simulink model "L5_2_G13_sim"  (R2024b)
settings: Solver=ode23tb  StartTime=0.0  StopTime=0.2  MaxStep=1/(fpwm_inv/200)  RelTol=1e-3
undefined symbols (not defined in the file): Cdc, deltafi, fac, Kii, Kivdc, Kpi, Kpvdc, Lfac, m_inv, Pac, Pdc, QCac, QLac, Rdc, Rdcmax, Udc, Vac, Vdcref, XLf
libraries: spsSeriesRLCBranchLib x6, spsThreePhaseVIMeasurementLib x3, spsCurrentMeasurementLib x2, spsabctodq0Lib x2, spsIdealSwitchLib x1, spsPLL3phLib x1, spsdq0toabcLib x1, spsPWMGenerator2LevelLib x1, spsMeanLib x1, spsPower3phInstantaneousLib x1, spsThreePhaseSourceLib x1, spsThreePhaseParallelRLCLoadLib x1
settings Model: Creator=franc  LastModifiedBy=franc

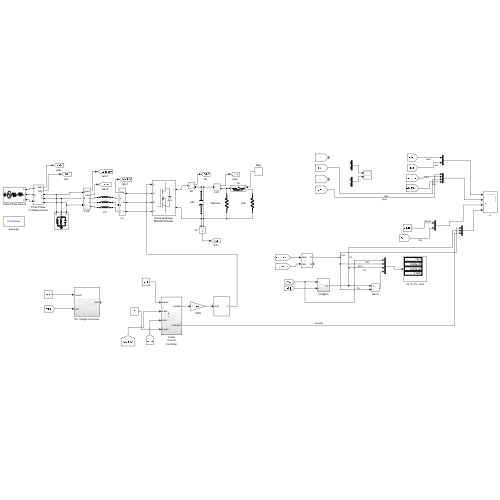
[thumbnail: Simulink's stored preview of the top-level diagram]
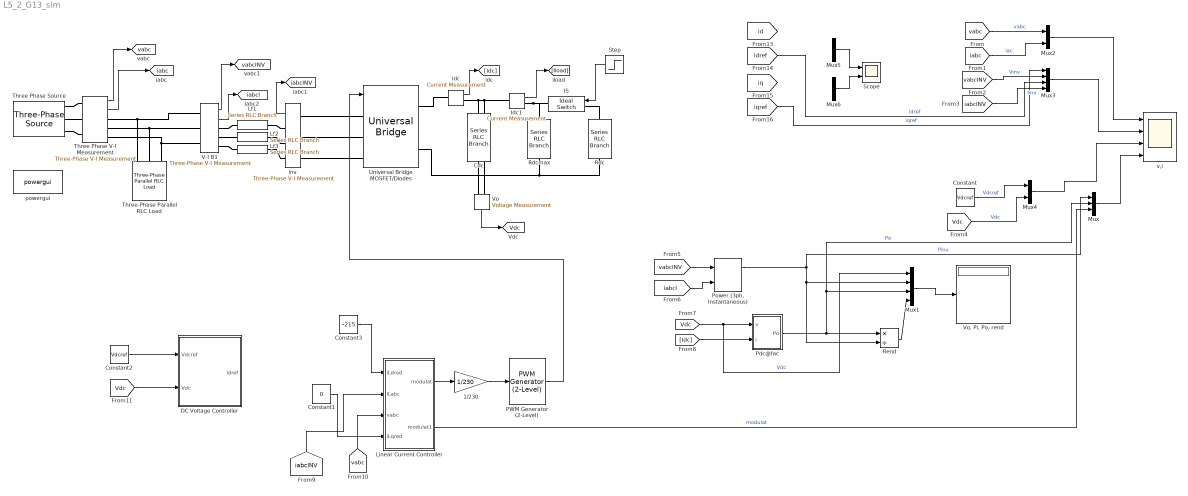
== system L5_2_G13_sim ==
  1/230 : Gain  Gain=1/230
  Cdc : spsSeriesRLCBranchLib/Series RLC Branch  LConnTagsString=__new0  RConnTagsString=__new0  BranchType=C  Resistance=1  Inductance=1e-3  SetiL0=off  InitialCurrent=0  Capacitance=Cdc  Setx0=on  InitialVoltage=0.95*Udc  Measurements=None
  Constant : Constant  Value=Vdcref
  Constant1 : Constant  Value=0
  Constant2 : Constant  Value=Vdcref
  Constant3 : Constant  Value=-215
  DC Voltage Controller : Subsystem
  IS : spsIdealSwitchLib/Ideal Switch  Ron=0.001  Lon=0  IC=0  Rs=1e5  Cs=inf  Measurements=off
  Idc : spsCurrentMeasurementLib/Current Measurement  PhasorSimulation=off  OutputType=Complex  PSBequivalent=0
  Idc1 : spsCurrentMeasurementLib/Current Measurement  PhasorSimulation=off  OutputType=Complex  PSBequivalent=0
  Lf1 : spsSeriesRLCBranchLib/Series RLC Branch  LConnTagsString=__new0  RConnTagsString=__new0  BranchType=L  Resistance=1  Inductance=Lfac  SetiL0=off  InitialCurrent=0  Capacitance=1e-6  Setx0=off  InitialVoltage=0  Measurements=None
  Lf2 : spsSeriesRLCBranchLib/Series RLC Branch  LConnTagsString=__new0  RConnTagsString=__new0  BranchType=L  Resistance=1  Inductance=Lfac  SetiL0=off  InitialCurrent=0  Capacitance=1e-6  Setx0=off  InitialVoltage=0  Measurements=None
  Lf3 : spsSeriesRLCBranchLib/Series RLC Branch  LConnTagsString=__new0  RConnTagsString=__new0  BranchType=L  Resistance=1  Inductance=Lfac  SetiL0=off  InitialCurrent=0  Capacitance=1e-6  Setx0=off  InitialVoltage=0  Measurements=None
  Linear Current Controller : Subsystem
  Mux : Mux  Inputs=3
  Mux1 : Mux
  Mux{2,4..6} (4 alike) : Mux  Inputs=2
  Mux3 : Mux
  PWM Generator (2-Level) : spsPWMGenerator2LevelLib/PWM Generator (2-Level)  ModulatorType=Three-phase bridge (6 pulses)  ModulatorMode=Unsynchronized  Fc=fpwm_inv  Pc=90  nF=27  MinMax="[ -1  1 ]"  SamplingTechnique=Asymmetrical regular (double edge)  ModulatingSignals=off  m=m_inv  Freq=fac  Phase=deltafi*180/pi  Ts=0  ShowCarrierOutport=off
  Pdc@fac : Subsystem
  "Power (3ph, Instantaneous)" : spsPower3phInstantaneousLib/Power (3ph, Instantaneous)
  Rdc : spsSeriesRLCBranchLib/Series RLC Branch  LConnTagsString=__new0  RConnTagsString=__new0  BranchType=R  Resistance=Rdc  Inductance=1e-3  SetiL0=off  InitialCurrent=0  Capacitance=1e-6  Setx0=off  InitialVoltage=0  Measurements=None
  Rdcmax : spsSeriesRLCBranchLib/Series RLC Branch  LConnTagsString=__new0  RConnTagsString=__new0  BranchType=R  Resistance=Rdcmax  Inductance=1e-3  SetiL0=off  InitialCurrent=0  Capacitance=1e-6  Setx0=off  InitialVoltage=0  Measurements=None
  Rend : Product  Inputs=*/
  Scope : Scope  NumInputPorts=2
  "Step " : Step  Time=0.06  SampleTime=0
  Three Phase V-I Measurement : spsThreePhaseVIMeasurementLib/Three-Phase V-I Measurement  VoltageMeasurement=phase-to-ground  SetLabelV=off  LabelV=Vabc  Vpu=off  VpuLL=off  CurrentMeasurement=yes  SetLabelI=off  LabelI=Iabc  Ipu=off  Pbase=100e6  Vbase=500e3  OutputType=Complex  PhasorSimulation=off  PSBequivalent=0
  Three Phase Source : spsThreePhaseSourceLib/Three-Phase Source  InternalConnection=Yg  VoltagePhases=off  Voltage=Vac*sqrt(3)  PhaseAngle=0  Voltage_phases=[25e3 25e3 25e3]/sqrt(3)  PhaseAngles_phases=[0 -120 +120]  Frequency=fac  NonIdealSource=on  SpecifyImpedance=on  Resistance=0.8929  Inductance=16.58e-3  ShortCircuitLevel=Scc  BaseVoltage=Vac*sqrt(3)  XRratio=X_R  BusType=swing  Pref=10e3  Qref=0  Prefabc=[10e3, 10e3, 10e3]  Qrefabc=[0, 0, 0]  Qmin=-inf  Qmax=inf
  Three-Phase Parallel RLC Load : spsThreePhaseParallelRLCLoadLib/Three-Phase Parallel RLC Load  LConnTagsString=A|B|C  Configuration=Y (grounded)  NominalVoltage=Vac*sqrt(3)  Vabc=[1e3 1e3 1e3]  Vabcp=[1e3 1e3 1e3]  NominalFrequency=fac  UnbalancedPower=off  ActivePower=Pac*3  InductivePower=QLac*3  CapacitivePower=QCac*3  Pabc=[10e3 9e3 11e3]  QLabc=[100 90 110]  QCabc=[100 90 110]  Pabcp=[10e3 9e3 11e3]  QLabcp=[100 90 110]  QCabcp=[100 90 110]  Measurements=None  LoadType=constant Z
  Universal Bridge MOSFET/Diodes : spsUniversalBridgeLib/Universal Bridge  Arms=3  SnubberResistance=Rs  SnubberCapacitance=inf  Device=MOSFET / Diodes  Ron=Ron  Lon=0  ForwardVoltages="[  0  0  ]"  ForwardVoltage=0  GTOparameters=[ 10e-6 , 20e-6 ]  IGBTparameters=[ 1e-6 , 2e-6 ]  Measurements=None  Measurements_2=None  converterType=Rectifier
  V-I B1 : spsThreePhaseVIMeasurementLib/Three-Phase V-I Measurement  VoltageMeasurement=phase-to-ground  SetLabelV=off  LabelV=Vabc  Vpu=off  VpuLL=off  CurrentMeasurement=yes  SetLabelI=off  LabelI=Iabc  Ipu=off  Pbase=100e6  Vbase=500e3  OutputType=Complex  PhasorSimulation=off  PSBequivalent=0
  Vo : spsVoltageMeasurementLib/Voltage Measurement  PhasorSimulation=off  OutputType=Complex  PSBequivalent=0
  "Vo, Pi, Po, rend" : Display
  inv : spsThreePhaseVIMeasurementLib/Three-Phase V-I Measurement  VoltageMeasurement=no  SetLabelV=off  LabelV=Vabc  Vpu=off  VpuLL=off  CurrentMeasurement=yes  SetLabelI=off  LabelI=Iabc  Ipu=off  Pbase=100e6  Vbase=500e3  OutputType=Complex  PhasorSimulation=off  PSBequivalent=0
  powergui : sps_lib/powergui  Priority=1  SimulationMode=Continuous  SampleTime=50e-6  frequency=60  Iterations=50  frequencyindice=50  Pbase=100e6  ErrMax=1e-4  UnitsV=kV  UnitsW=MW  buscounter=0  FunctionMessages=off  echomessages=off  EnableUseOfTLC=off  CurrentSourceSwitches=off  DisableSnubberDevices=off  DisableRonSwitches=off  DisableVfSwitches=off  DisplayEquations=off  AutomaticDiscreteSolvers=off  SolverType=Tustin/Backward Euler (TBE)  Interpol=off  ExternalGateDelay=off  methode=off  Ts=100  x0status=blocks  SPID=on  SwTol=0  HookPort=off  NonlinearTolerance=1e-4  nMaxIteration=100  ContinueOnMaxIteration=off  RestoreLinks=warning  ResistiveCurrentMeasurement=off  Frange=[0:2:500]  Ylog=off  Xlog=on  ShowGrid=off  save=off  variable=ZData  structure=0  ZoomFFT=off  StartTime=0.0  cycles=1  DisplayStyle=1  fundamental=60  FreqAxis=off  MaxFrequency=1000  frequencyindicesteady=1  RmsSteady=1  display=off
  v,i : Scope  NumInputPorts=4
  tag scope: Vdc=global, iabc=global, iabcINV=global, iabcl=global, vabc=global, vabcINV=global
  wires:
  Three Phase V-I Measurement/1 -> [vabc]
  Three Phase V-I Measurement/2 -> [iabc]
  V-I B1/1 -> [vabcINV]
  V-I B1/2 -> [iabcl]
  inv/1 -> [iabcINV]
  Vo/1 -> [Vdc]
  Idc/1 -> [Idc]
  Idc1/1 -> [Iload]
  "Step "/1 -> IS/1
  Rend/1 -> Mux1/4
  [Vdc] -> Pdc@fac/1(v), Mux1/1  "Vdc"
  Mux1/1 -> "Vo, Pi, Po, rend"/1
  [iabc] -> Mux2/2  "iac"
  [vabc] -> Mux2/1  "vabc"
  Mux2/1 -> v,i/1
  [vabcINV] -> Mux3/2  "Vinv"
  [iabcINV] -> Mux3/4  "Iinv"
  Mux3/1 -> v,i/2
  Constant/1 -> Mux4/1  "Vdcref"
  [Vdc] -> Mux4/2  "Vdc"
  Mux4/1 -> v,i/3
  Mux/1 -> v,i/4
  [iabcl] -> "Power (3ph, Instantaneous)"/2
  [vabcINV] -> "Power (3ph, Instantaneous)"/1
  "Power (3ph, Instantaneous)"/1 -> Mux/1, Rend/2, Mux1/2  "Pinv"
  [Idc] -> Pdc@fac/2(i)
  Pdc@fac/1(Po) -> Mux1/3, Mux/2, Rend/1  "Po"
  Linear Current Controller/1(modulat) -> 1/230/1
  [vabc] -> Linear Current Controller/3(vabc)
  [iabcINV] -> Linear Current Controller/2(iLabc)
  Constant1/1 -> Linear Current Controller/4(iLqred)
  [Vdc] -> DC Voltage Controller/2(Vdc)
  Constant2/1 -> DC Voltage Controller/1(Vdcref)
  PWM Generator (2-Level)/1 -> Universal Bridge MOSFET/Diodes/1
  Linear Current Controller/2(modulat1) -> Mux/3  "modulat"
  1/230/1 -> PWM Generator (2-Level)/1
  Mux5/1 -> Scope/1
  Mux6/1 -> Scope/2
  Constant3/1 -> Linear Current Controller/1(iLdred)
  [idref] -> Mux3/3  "idref"
  [iqref] -> Mux3/1  "iqref"
  connections:
  Three Phase Source/RConn1 -- Three Phase V-I Measurement/LConn1
  Three Phase Source/RConn2 -- Three Phase V-I Measurement/LConn2
  Three Phase Source/RConn3 -- Three Phase V-I Measurement/LConn3
  Three Phase V-I Measurement/RConn1 -- Three-Phase Parallel RLC Load/LConn1 -- V-I B1/LConn1
  Three Phase V-I Measurement/RConn2 -- Three-Phase Parallel RLC Load/LConn2 -- V-I B1/LConn2
  Three Phase V-I Measurement/RConn3 -- Three-Phase Parallel RLC Load/LConn3 -- V-I B1/LConn3
  V-I B1/RConn3 -- Lf3/LConn1
  V-I B1/RConn2 -- Lf2/LConn1
  V-I B1/RConn1 -- Lf1/LConn1
  Universal Bridge MOSFET/Diodes/RConn1 -- Idc/LConn1
  Idc/RConn1 -- Idc1/LConn1 -- Vo/LConn1 -- Cdc/LConn1
  Idc1/RConn1 -- Rdcmax/LConn1 -- IS/RConn1
  IS/LConn1 -- Rdc/LConn1
  Rdc/RConn1 -- Vo/LConn2 -- Cdc/RConn1 -- Universal Bridge MOSFET/Diodes/RConn2 -- Rdcmax/RConn1
  inv/LConn1 -- Universal Bridge MOSFET/Diodes/LConn1
  inv/LConn2 -- Universal Bridge MOSFET/Diodes/LConn2
  inv/LConn3 -- Universal Bridge MOSFET/Diodes/LConn3
  Lf3/RConn1 -- inv/RConn3
  Lf2/RConn1 -- inv/RConn2
  Lf1/RConn1 -- inv/RConn1

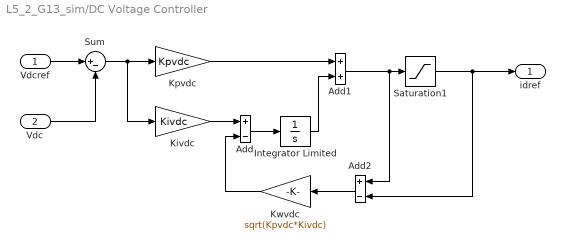
== system L5_2_G13_sim/DC Voltage Controller ==
  Vdcref : Inport
  Vdc : Inport  Port=2
  Add : Sum  Inputs=+-
  Add1 : Sum
  Add2 : Sum  Inputs=+-
  Integrator Limited : Integrator  LimitOutput=on  UpperSaturationLimit=1000  LowerSaturationLimit=-1000
  Kivdc : Gain  Gain=Kivdc
  Kpvdc : Gain  Gain=Kpvdc
  Kwvdc : Gain  Gain=sqrt(Kpvdc*Kivdc)
  Saturation1 : Saturate  UpperLimit=1000  LowerLimit=-1000
  Sum : Sum  Inputs=|+-
  idref : Outport
  wires:
  Vdcref/1 -> Sum/1
  Vdc/1 -> Sum/2
  Sum/1 -> Kivdc/1, Kpvdc/1
  Kivdc/1 -> Add/1
  Kpvdc/1 -> Add1/1
  Integrator Limited/1 -> Add1/2
  Add/1 -> Integrator Limited/1
  Add1/1 -> Add2/1, Saturation1/1
  Kwvdc/1 -> Add/2
  Add2/1 -> Kwvdc/1
  Saturation1/1 -> Add2/2, idref/1

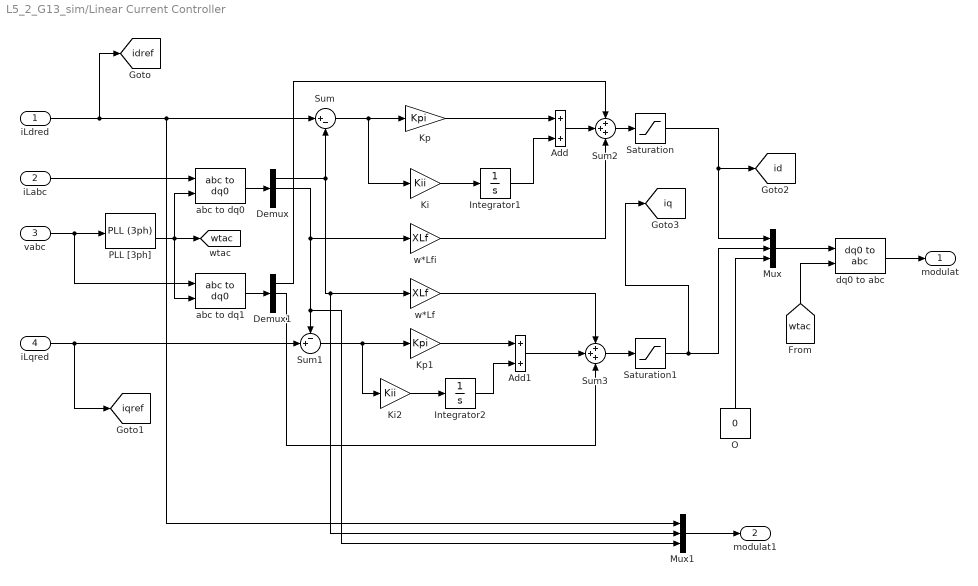
== system L5_2_G13_sim/Linear Current Controller ==
  iLdred : Inport
  iLabc : Inport  Port=2
  vabc : Inport  Port=3
  iLqred : Inport  Port=4
  Add : Sum
  Add1 : Sum
  Demux : Demux  Outputs=3
  Demux1 : Demux  Outputs=3
  Integrator1 : Integrator  LimitOutput=on  UpperSaturationLimit=300  LowerSaturationLimit=-300
  Integrator2 : Integrator  LimitOutput=on  UpperSaturationLimit=300  LowerSaturationLimit=-300
  Ki : Gain  Gain=Kii
  Ki2 : Gain  Gain=Kii
  Kp : Gain  Gain=Kpi
  Kp1 : Gain  Gain=Kpi
  Mux : Mux  Inputs=3
  Mux1 : Mux  Inputs=3
  O : Constant  Value=0
  PLL [3ph] : spsPLL3phLib/PLL (3ph)  Fmin=45  Par_Init=[0, 50]  ParK=[180, 3200, 1]  TcD=1e-4  MaxRateChangeFreq=12  FilterCutOffFreq=25  Ts=0  AGC=on
  Saturation : Saturate  UpperLimit=300  LowerLimit=-300
  Saturation1 : Saturate  UpperLimit=300  LowerLimit=-300
  Sum : Sum  Inputs=|+-
  Sum1 : Sum  Inputs=-+|
  Sum2 : Sum  Inputs=+++
  Sum3 : Sum  Inputs=+++
  abc to dq0 : spsabctodq0Lib/abc to dq0  Alignment=90 degrees behind phase A axis
  abc to dq1 : spsabctodq0Lib/abc to dq0  Alignment=90 degrees behind phase A axis
  dq0 to abc : spsdq0toabcLib/dq0 to abc  Alignment=90 degrees behind phase A axis
  w*Lf : Gain  Gain=XLf
  w*Lfi : Gain  Gain=XLf
  modulat : Outport
  modulat1 : Outport  Port=2
  tag scope: id=global, idref=global, iq=global, iqref=global, wtac=global
  wires:
  vabc/1 -> abc to dq1/1, PLL [3ph]/1
  iLabc/1 -> abc to dq0/1
  PLL [3ph]/2 -> abc to dq1/2, [wtac], abc to dq0/2
  iLdred/1 -> [idref], Mux1/1, Sum/1
  abc to dq0/1 -> Demux/1
  abc to dq1/1 -> Demux1/1
  Sum/1 -> Ki/1, Kp/1
  Demux/1 -> Sum/2, w*Lf/1, Mux1/2
  Sum1/1 -> Ki2/1, Kp1/1
  Ki2/1 -> Integrator2/1
  Ki/1 -> Integrator1/1
  Kp/1 -> Add/1
  Integrator1/1 -> Add/2
  Kp1/1 -> Add1/1
  Integrator2/1 -> Add1/2
  Add/1 -> Sum2/2
  Add1/1 -> Sum3/2
  Demux1/2 -> Sum3/3
  w*Lf/1 -> Sum3/1
  Sum3/1 -> Saturation1/1
  w*Lfi/1 -> Sum2/3
  Sum2/1 -> Saturation/1
  Demux1/1 -> Sum2/1
  Saturation1/1 -> [iq], Mux/2
  O/1 -> Mux/3
  Mux/1 -> dq0 to abc/1
  [wtac] -> dq0 to abc/2
  dq0 to abc/1 -> modulat/1
  Mux1/1 -> modulat1/1
  Demux/2 -> Mux1/3, Sum1/1, w*Lfi/1
  iLqred/1 -> [iqref], Sum1/2
  Saturation/1 -> [id], Mux/1

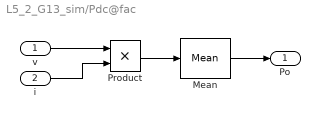
== system L5_2_G13_sim/Pdc@fac ==
  v : Inport
  i : Inport  Port=2
  Mean : spsMeanLib/Mean  Freq=fac*10  Vinit=Pdc/2  Ts=0
  Product : Product
  Po : Outport
  wires:
  Mean/1 -> Po/1
  i/1 -> Product/2
  v/1 -> Product/1
  Product/1 -> Mean/1
